simulink model "hill_type_muscle_model"  (R2013a)
settings: Solver=ode45  StartTime=0.0  StopTime=10.0  RelTol=1e-3
libraries: nesl_utility x4
settings Model: Creator=Administrator  LastModifiedBy=Administrator

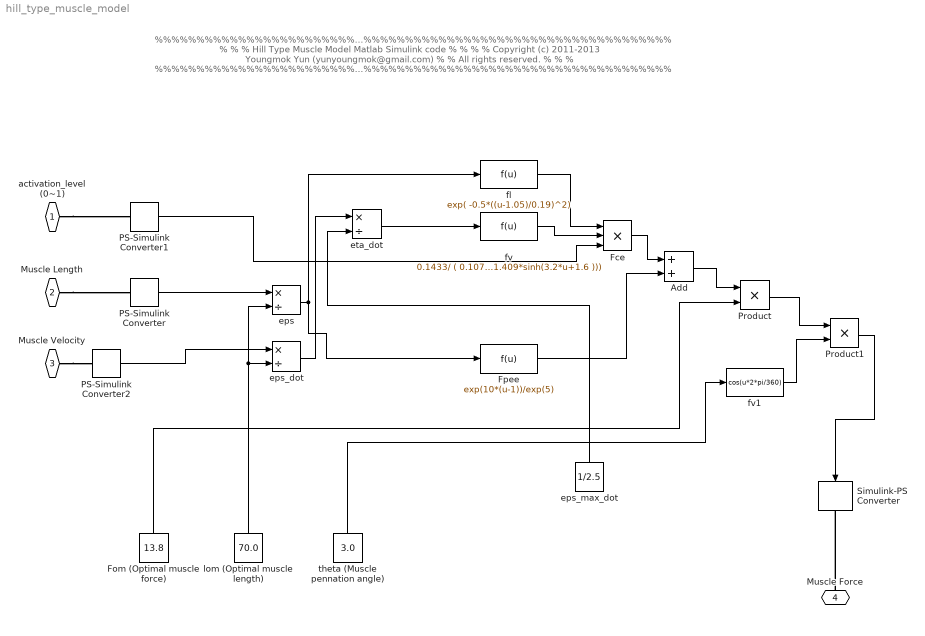
== system hill_type_muscle_model ==
  note: %%%%%%%%%%%%%%%%%%%%%%%%%%%%%%%%%%%%%%%%%%%%%%%%%%%%%%%%%%%%%%%%%%%%%%%%%%%%
      | %                                                                          %
      | %                   Hill Type Muscle Model Matlab Simulink code                     %
      | %                                                                          %
      | %  Copyright (c) 2011-2013 Youngmok Yun (yunyoungmok@gmail.com)            %
      | %                                          All rights reserved.            %
      | %                                                                          %
      | %%%%%%%%%%%%%%%%%%%%%%%%%%%%%%%%%%%%%%%%%%%%%%%%%%%%%%%%%%%%%%%%%%%%%%%%%%%%
  Add : Sum
  Fce : Product  Inputs=3
  Fom (Optimal muscle force) : Constant  Value=13.8
  Fpee : Fcn  Expr=exp(10*(u-1))/exp(5)
  PS-Simulink Converter : nesl_utility/PS-Simulink Converter  PhysicalDomain=network_engine_domain  SubClassName=ps_output  LeftPortType=input  RightPortType=output  PseudoPeriodic=off  Frequencies=[]  Unit=1  AffineConversion=off
  PS-Simulink Converter1 : nesl_utility/PS-Simulink Converter  PhysicalDomain=network_engine_domain  SubClassName=ps_output  LeftPortType=input  RightPortType=output  PseudoPeriodic=off  Frequencies=[]  Unit=1  AffineConversion=off
  PS-Simulink Converter2 : nesl_utility/PS-Simulink Converter  PhysicalDomain=network_engine_domain  SubClassName=ps_output  LeftPortType=input  RightPortType=output  PseudoPeriodic=off  Frequencies=[]  Unit=1  AffineConversion=off
  Product : Product
  Product1 : Product
  Simulink-PS Converter : nesl_utility/Simulink-PS Converter  PhysicalDomain=network_engine_domain  SubClassName=ps_input  LeftPortType=input  RightPortType=output  PseudoPeriodic=off  Frequencies=[]  NoiseDistribution=none  NoiseParameters=[]  Unit=1  AffineConversion=off  InputFiltering=off  SimscapeFilterOrder=1  InputFilterTimeConstant=0.001  UdotUserProvided=1
  eps : Product  Inputs=*/
  eps_dot : Product  Inputs=*/
  eps_max_dot : Constant  Value=1/2.5
  eta_dot : Product  Inputs=*/
  fl : Fcn  Expr=exp( -0.5*((u-1.05)/0.19)^2)
  fv : Fcn  Expr=0.1433/ ( 0.1074+exp(-1.409*sinh(3.2*u+1.6 )))
  fv1 : Fcn  Expr=cos(u*2*pi/360)
  lom (Optimal muscle length) : Constant  Value=70.0
  theta (Muscle pennation angle) : Constant  Value=3.0
  activation_level (0~1) : PMIOPort  Port=1  Side=Left
  Muscle Length : PMIOPort  Port=2  Side=Right
  Muscle Velocity : PMIOPort  Port=3  Side=Left
  Muscle Force : PMIOPort  Port=4  Side=Right
  wires:
  lom (Optimal muscle length)/1 -> eps_dot/2, eps/2
  eps_dot/1 -> eta_dot/1
  eps_max_dot/1 -> eta_dot/2
  eps/1 -> fl/1, Fpee/1
  eta_dot/1 -> fv/1
  fl/1 -> Fce/1
  fv/1 -> Fce/2
  Fpee/1 -> Add/2
  Add/1 -> Product/1
  Fom (Optimal muscle force)/1 -> Product/2
  theta (Muscle pennation angle)/1 -> fv1/1
  Product/1 -> Product1/1
  fv1/1 -> Product1/2
  Product1/1 -> Simulink-PS Converter/1
  Fce/1 -> Add/1
  PS-Simulink Converter1/1 -> Fce/3
  PS-Simulink Converter/1 -> eps/1
  PS-Simulink Converter2/1 -> eps_dot/1
  connections:
  Muscle Length/RConn1 -- PS-Simulink Converter/LConn1
  Muscle Velocity/RConn1 -- PS-Simulink Converter2/LConn1
  activation_level (0~1)/RConn1 -- PS-Simulink Converter1/LConn1
  Muscle Force/RConn1 -- Simulink-PS Converter/RConn1
